simulink library "INT_FuelT_DD"  (R2016b)
settings: Solver=VariableStepAuto  StartTime=0.0  StopTime=10.0  RelTol=1e-3
settings Model: Creator=Administrator  LastModifiedBy=Administrator

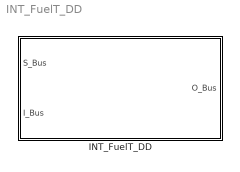
== system INT_FuelT_DD ==
  INT_FuelT_DD : Subsystem

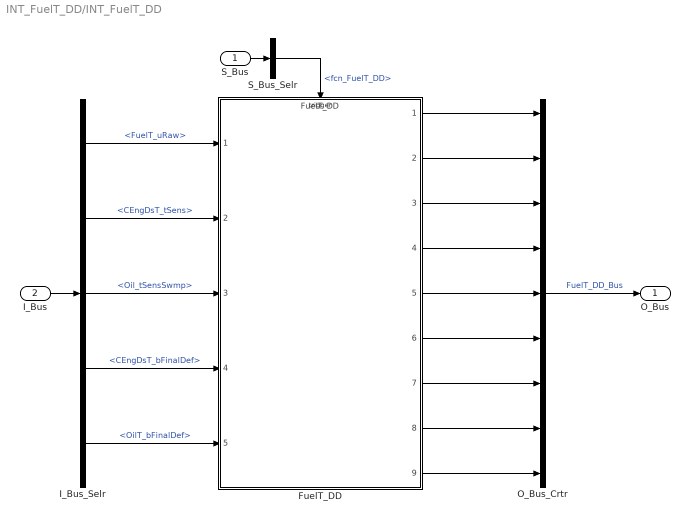
== system INT_FuelT_DD/INT_FuelT_DD ==
  S_Bus : Inport
  I_Bus : Inport  Port=2
  FuelT_DD : ModelReference  ModelNameDialog=FuelT_DD  SimulationMode=Normal  ModelReferenceVersion=1.3  TriggerPortName=function  TriggerPortTriggerType=function-call  TriggerPortStatesWhenEnabling=held
  I_Bus_Selr : BusSelector  OutputSignals=FuelT_uRaw,CEngDsT_tSens,Oil_tSensSwmp,CEngDsT_bFinalDef,OilT_bFinalDef
  O_Bus_Crtr : BusCreator  Inputs=9
  S_Bus_Selr : BusSelector  OutputSignals=fcn_FuelT_DD
  O_Bus : Outport
  wires:
  S_Bus_Selr/1 -> FuelT_DD/Trigger  "<fcn_FuelT_DD>"
  S_Bus/1 -> S_Bus_Selr/1
  I_Bus/1 -> I_Bus_Selr/1
  I_Bus_Selr/1 -> FuelT_DD/1  "<FuelT_uRaw>"
  I_Bus_Selr/2 -> FuelT_DD/2  "<CEngDsT_tSens>"
  I_Bus_Selr/3 -> FuelT_DD/3  "<Oil_tSensSwmp>"
  I_Bus_Selr/4 -> FuelT_DD/4  "<CEngDsT_bFinalDef>"
  I_Bus_Selr/5 -> FuelT_DD/5  "<OilT_bFinalDef>"
  O_Bus_Crtr/1 -> O_Bus/1  "FuelT_DD_Bus"
  FuelT_DD/1 -> O_Bus_Crtr/1
  FuelT_DD/2 -> O_Bus_Crtr/2
  FuelT_DD/3 -> O_Bus_Crtr/3
  FuelT_DD/4 -> O_Bus_Crtr/4
  FuelT_DD/5 -> O_Bus_Crtr/5
  FuelT_DD/6 -> O_Bus_Crtr/6
  FuelT_DD/7 -> O_Bus_Crtr/7
  FuelT_DD/8 -> O_Bus_Crtr/8
  FuelT_DD/9 -> O_Bus_Crtr/9
